simulink model "combined"  (R2015b)
settings: Solver=VariableStepAuto  StartTime=0.0  StopTime=10.0  RelTol=1e-3
values from neighbouring files (symbols this model uses):
  l1_val = 500e-4    (= 0.05)    [CurrentSourceController.m]    (also in main.m = 4.8e-07)
  r_val = 1    [CurrentSourceController.m]    (also in VoltageSourceController.m; main.m)
  rl1_val = 0.0002    [CurrentSourceController.m]    (also in main.m)
  Vd_val = 100    [CurrentSourceController.m]    (also in VoltageSourceController.m = 8; main.m = 110)
undefined symbols (not defined in the file or in its folder): Ac, c_val, den_c1, fs, l_val, num_c1
libraries: powerlib x19, simulink x2, simulink_extras x2, powerlib_meascontrol x1
settings Model: Creator=Akshay  LastModifiedBy=Akshay

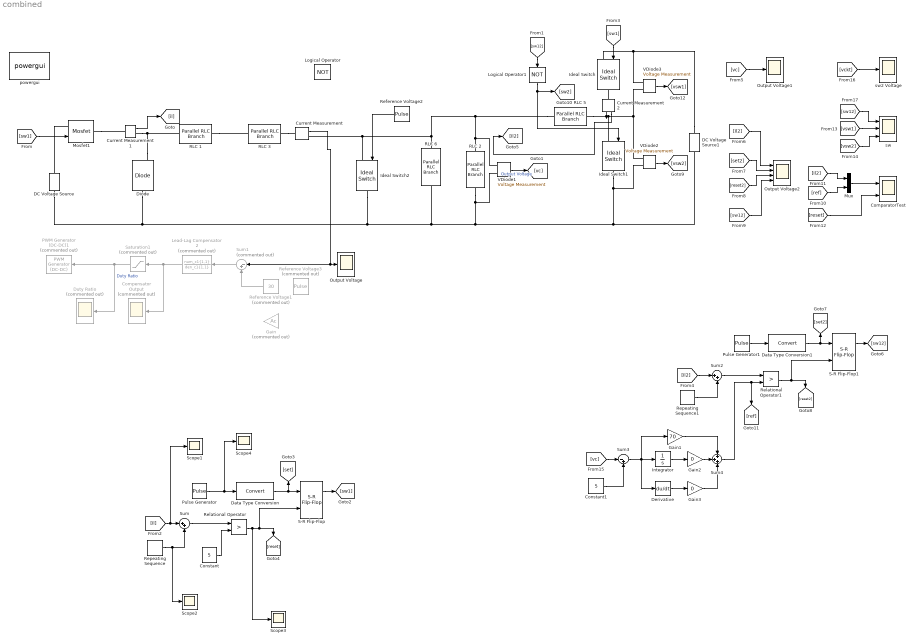
== system combined ==
  " RLC 1" : powerlib/Elements/Parallel RLC Branch  LConnTagsString=a  RConnTagsString=__new0  BranchType=R  Resistance=rl1_val  Inductance=5e-6  SetiL0=off  InitialCurrent=0  Capacitance=0.3e-6  Setx0=off  InitialVoltage=0  Measurements=None
  " RLC 2" : powerlib/Elements/Parallel RLC Branch  LConnTagsString=a  RConnTagsString=__new0  BranchType=C  Resistance=1  Inductance=1e-3  SetiL0=off  InitialCurrent=0  Capacitance=c_val  Setx0=off  InitialVoltage=50  Measurements=None
  " RLC 3" : powerlib/Elements/Parallel RLC Branch  LConnTagsString=a  RConnTagsString=__new0  BranchType=L  Resistance=50  Inductance=l1_val  SetiL0=off  InitialCurrent=100  Capacitance=0.3e-6  Setx0=off  InitialVoltage=0  Measurements=None
  " RLC 5" : powerlib/Elements/Parallel RLC Branch  LConnTagsString=a  RConnTagsString=__new0  BranchType=L  Resistance=50  Inductance=l_val  SetiL0=on  InitialCurrent=0  Capacitance=0.3e-6  Setx0=off  InitialVoltage=0  Measurements=None
  " RLC 6" : powerlib/Elements/Parallel RLC Branch  LConnTagsString=a  RConnTagsString=__new0  BranchType=R  Resistance=r_val  Inductance=1e-3  SetiL0=off  InitialCurrent=0  Capacitance=0.1e-6  Setx0=off  InitialVoltage=0  Measurements=None
  ComparatorTest : Scope  NumInputPorts=2
  Compensator Output : Scope  Commented=on
  Constant : Constant  Value=5
  Constant1 : Constant  Value=5
  Current Measurement : powerlib/Measurements/Current Measurement  PhasorSimulation=off  OutputType=Complex  PSBequivalent=0
  Current Measurement1 : powerlib/Measurements/Current Measurement  PhasorSimulation=off  OutputType=Complex  PSBequivalent=0
  Current Measurement2 : powerlib/Measurements/Current Measurement  PhasorSimulation=off  OutputType=Complex  PSBequivalent=0
  DC Voltage Source : powerlib/Electrical Sources/DC Voltage Source  Amplitude=Vd_val  Measurements=Voltage
  DC Voltage Source1 : powerlib/Electrical Sources/DC Voltage Source  Amplitude=Vd_val  Measurements=Voltage
  Data Type Conversion : DataTypeConversion
  Data Type Conversion1 : DataTypeConversion
  Derivative : Derivative
  Diode : powerlib/Power Electronics/Diode  Ron=0.001  Lon=0  Vf=0.8  IC=0  UseSnubber=off  Rs=500  Cs=250e-9  Measurements=on
  Duty Ratio : Scope  Commented=on
  Gain : Gain  Commented=on  Gain=Ac
  Gain1 : Gain  Gain=70
  Gain2 : Gain  Gain=0
  Gain3 : Gain  Gain=0
  Ideal Switch : powerlib/Power Electronics/Ideal Switch  Ron=1e-7  Lon=0  IC=0  Rs=inf  Cs=inf  Measurements=off
  Ideal Switch1 : powerlib/Power Electronics/Ideal Switch  Ron=1e-7  Lon=0  IC=1  Rs=inf  Cs=inf  Measurements=off
  Ideal Switch2 : powerlib/Power Electronics/Ideal Switch  Ron=1e-7  Lon=0  IC=1  Rs=inf  Cs=inf  Measurements=off
  Integrator : Integrator
  Lead-Lag Compensator2 : TransferFcn  Commented=on  Numerator=num_c1{1,1}  Denominator=den_c1{1,1}
  Logical Operator : Logic  Operator=NOT  AllPortsSameDT=off  OutDataTypeStr=boolean
  Logical Operator1 : Logic  Operator=NOT  AllPortsSameDT=off  OutDataTypeStr=boolean
  Mosfet1 : powerlib/Power Electronics/Mosfet  Ron=0.00001  Lon=0  Rd=0.0000000000001  Vfd=0  IC=0  Rs=1e5  Cs=inf  Measurements=off
  Mux : Mux  Inputs=2
  Output Voltage : Scope
  Output Voltage1 : Scope
  Output Voltage2 : Scope  NumInputPorts=4
  PWM Generator (DC-DC)1 : powerlib_meascontrol/Pulse & Signal Generators/PWM Generator (DC-DC)  Commented=on  Fsw=1e6  Ts=0
  Pulse Generator : DiscretePulseGenerator  PulseType=Time based  Period=1/fs  PulseWidth=5
  Pulse Generator1 : DiscretePulseGenerator  PulseType=Time based  Period=1/fs  PulseWidth=5
  Reference Voltage1 : Constant  Commented=on  Value=30
  Reference Voltage2 : DiscretePulseGenerator  PulseType=Time based  Period=10/fs  PulseWidth=6  PhaseDelay=1/fs
  Reference Voltage3 : DiscretePulseGenerator  Commented=on  PulseType=Time based  Amplitude=70  Period=180e-6  PulseWidth=6
  Relational Operator : RelationalOperator  Operator=>  OutDataTypeStr=boolean
  Relational Operator1 : RelationalOperator  Operator=>  OutDataTypeStr=boolean
  Repeating Sequence : simulink/Sources/Repeating Sequence  rep_seq_t=[0 1/fs]  rep_seq_y=[0 0]
  Repeating Sequence1 : simulink/Sources/Repeating Sequence  rep_seq_t=[0 1/fs]  rep_seq_y=[0 0]
  S-R Flip-Flop : simulink_extras/Flip Flops/S-R Flip-Flop  initial_condition=0
  S-R Flip-Flop1 : simulink_extras/Flip Flops/S-R Flip-Flop  initial_condition=0
  Saturation1 : Saturate  Commented=on  UpperLimit=1  LowerLimit=0  ZeroCross=off
  Scope{1..4} (4 alike) : Scope
  Sum : Sum  Inputs=|++
  Sum1 : Sum  Commented=on  Inputs=|-+
  Sum2 : Sum  Inputs=|++
  Sum3 : Sum  Inputs=|-+
  Sum4 : Sum  Inputs=+++
  VDiode1 : powerlib/Measurements/Voltage Measurement  PhasorSimulation=off  OutputType=Complex  PSBequivalent=0
  VDiode2 : powerlib/Measurements/Voltage Measurement  PhasorSimulation=off  OutputType=Complex  PSBequivalent=0
  VDiode3 : powerlib/Measurements/Voltage Measurement  PhasorSimulation=off  OutputType=Complex  PSBequivalent=0
  powergui : powerlib/powergui  Priority=1  SimulationMode=Continuous  SolverType=Backward Euler  SampleTime=5e-07  frequency=60  SPID=on  DisableSnubberDevices=off  DisableRonSwitches=off  DisableVfSwitches=off  SwTol=0  DisplayEquations=off  Interpol=off  ExternalGateDelay=off  methode=off  Ts=0  FunctionMessages=off  echomessages=off  HookPort=off  EnableUseOfTLC=off  x0status=zero  frequencyindice=0  Pbase=100e6  ErrMax=1e-4  Iterations=50  UnitsV=kV  UnitsW=MW  buscounter=0  RestoreLinks=warning  ResistiveCurrentMeasurement=off  Frange=[0:2:500]  Ylog=off  Xlog=on  ShowGrid=off  save=off  variable=ZData  structure=ScopeData  ZoomFFT=off  StartTime=0.0  cycles=5  DisplayStyle=2  fundamental=50  FreqAxis=off  MaxFrequency=50000  frequencyindicesteady=1  RmsSteady=1  display=off
  sw : Scope  NumInputPorts=3
  sw2 Voltage : Scope
  wires:
  Current Measurement/1 -> Sum1/1, Output Voltage/1
  Saturation1/1 -> Duty Ratio/1, PWM Generator (DC-DC)1/1  "Duty Ratio"
  Reference Voltage1/1 -> Sum1/2
  Lead-Lag Compensator2/1 -> Compensator Output/1, Saturation1/1
  Sum1/1 -> Lead-Lag Compensator2/1
  Pulse Generator/1 -> Scope4/1, Data Type Conversion/1
  Data Type Conversion/1 -> S-R Flip-Flop/1, [set]
  Relational Operator/1 -> Scope3/1, S-R Flip-Flop/2, [reset]
  S-R Flip-Flop/1 -> [sw1]
  [il] -> Scope1/1, Sum/1
  Repeating Sequence/1 -> Scope2/1, Sum/2
  Sum/1 -> Relational Operator/1
  Current Measurement1/1 -> [il]
  Constant/1 -> Relational Operator/2
  [sw1] -> Mosfet1/1
  VDiode1/1 -> [vc]  "Output Voltage"
  Current Measurement2/1 -> [il2]
  Pulse Generator1/1 -> Data Type Conversion1/1
  Data Type Conversion1/1 -> S-R Flip-Flop1/1, [set2]
  [sw12] -> Logical Operator1/1
  Relational Operator1/1 -> S-R Flip-Flop1/2, [reset2]
  [vc] -> Output Voltage1/1
  [il2] -> Output Voltage2/1
  [set2] -> Output Voltage2/2
  [reset2] -> Output Voltage2/3
  [sw12] -> Output Voltage2/4
  VDiode2/1 -> [vsw2]
  [vckt] -> sw2 Voltage/1
  [sw12] -> sw/1
  S-R Flip-Flop1/1 -> [sw12]
  Logical Operator1/1 -> [sw2], Ideal Switch1/1
  [sw1] -> Ideal Switch/1
  [il2] -> Mux/1
  [ref] -> Mux/2
  Mux/1 -> ComparatorTest/1
  [reset] -> ComparatorTest/2
  VDiode3/1 -> [vsw1]
  [vsw2] -> sw/3
  [vsw1] -> sw/2
  [il2] -> Sum2/1
  Repeating Sequence1/1 -> Sum2/2
  Sum2/1 -> Relational Operator1/1
  [vc] -> Sum3/1
  Constant1/1 -> Sum3/2
  Sum3/1 -> Derivative/1, Gain1/1, Integrator/1
  Integrator/1 -> Gain2/1
  Gain2/1 -> Sum4/2
  Gain1/1 -> Sum4/1
  Sum4/1 -> Relational Operator1/2, [ref]
  Derivative/1 -> Gain3/1
  Gain3/1 -> Sum4/3
  Reference Voltage2/1 -> Ideal Switch2/1
  connections:
  Diode/RConn1 -- " RLC 1"/LConn1 -- Current Measurement1/RConn1
  " RLC 1"/RConn1 -- " RLC 3"/LConn1
  DC Voltage Source/RConn1 -- Mosfet1/LConn1
  " RLC 3"/RConn1 -- Current Measurement/LConn1
  Mosfet1/RConn1 -- Current Measurement1/LConn1
  Ideal Switch1/LConn1 -- VDiode3/LConn2 -- VDiode2/LConn1 -- " RLC 5"/RConn1 -- Current Measurement2/RConn1
  Diode/LConn1 -- DC Voltage Source/LConn1 -- Ideal Switch2/RConn1 -- " RLC 6"/RConn1 -- Ideal Switch1/RConn1 -- VDiode2/LConn2 -- DC Voltage Source1/LConn1 -- " RLC 2"/RConn1 -- VDiode1/LConn2
  " RLC 5"/LConn1 -- Ideal Switch2/LConn1 -- Current Measurement/RConn1 -- " RLC 6"/LConn1 -- " RLC 2"/LConn1 -- VDiode1/LConn1
  DC Voltage Source1/RConn1 -- Ideal Switch/LConn1 -- VDiode3/LConn1
  Current Measurement2/LConn1 -- Ideal Switch/RConn1
